simulink model "model3_19b"  (R2019b)
settings: Solver=VariableStepAuto  StartTime=0.0  StopTime=200  RelTol=1e-3
model workspace (MAT data in the model file):
  x2xx = 0
values from neighbouring files (symbols this model uses):
  axle_rate_limit = 1    [call_AFG4hil_s1v1.m]
  Kad = 0.0    (= 0)    [call_AFG4hil_s1v1.m]
  Kai = 0.05    [call_AFG4hil_s1v1.m]
  Kap = 0.1    [call_AFG4hil_s1v1.m]
  KDspd = 0.1    [call_AFG4hil_s1v1.m]    (also in call_AFG_s1v1.m = 0)
  KIspd = 0.1    [call_AFG4hil_s1v1.m]    (also in call_AFG_s1v1.m = 0)
  KPspd = 10    [call_AFG4hil_s1v1.m]    (also in call_AFG_s1v1.m = 20)
  Lspd = -7    [call_AFG4hil_s1v1.m]
  Nspd = 10    [call_AFG4hil_s1v1.m]
  Tmc = 0.02    [call_AFG4hil_s1v1.m]    (also in call_AFG_s1v1.m = 0.01)
  TRACK = temptrack    [article.m]    (also in calculate_offtrack.m; call_AFG4hil_s1v1.m = trackgen4(2,50); call_AFG_s1v1.m = trackgen4(2,50); tracktest.m)
  Tst = 0.05    [call_AFG4hil_s1v1.m]    (also in call_AFG_s1v1.m = 0.02)
  Uspd = 5    [call_AFG4hil_s1v1.m]
  vconst = 15*kph    (= 4.16666666667)    [call_AFG4hil_s1v1.m]    (also in call_AFG_s1v1.m = 5.55555555556)
undefined symbols (not defined in the file or in its folder): PARSa, PARSu, Q0
libraries: simulink x2
settings Model: Creator=DJW  LastModifiedBy=14668

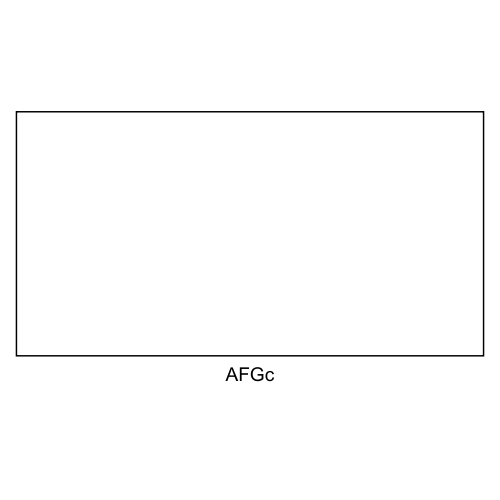
[thumbnail: Simulink's stored preview of the top-level diagram]
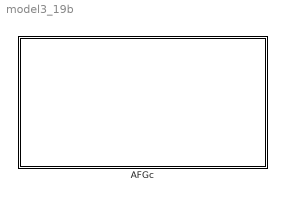
== system model3_19b ==
  AFGc : Subsystem

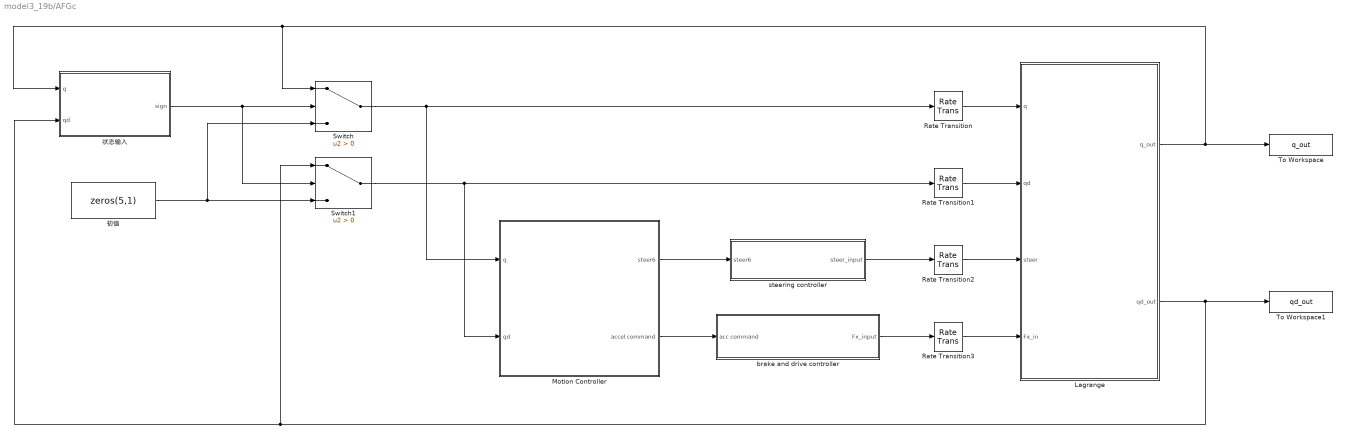
== system model3_19b/AFGc ==
  " Motion Controller" : Subsystem  SystemSampleTime=Tmc
  Lagrange : Subsystem
  Rate Transition{,1..3} (4 alike) : RateTransition
  Switch : Switch  Criteria=u2 > Threshold
  Switch1 : Switch  Criteria=u2 > Threshold
  To Workspace : ToWorkspace  VariableName=q_out  SampleTime=-1
  To Workspace1 : ToWorkspace  VariableName=qd_out  SampleTime=-1
  brake and drive controller : Subsystem
  steering controller : Subsystem
  初值 : Constant  Value=zeros(5,1)
  状态输入 : MATLAB Function  TreatAsAtomicUnit=on
  wires:
  " Motion Controller"/1(steer6) -> steering controller/1(steer6)
  " Motion Controller"/2(accel command) -> brake and drive controller/1(acc command)
  steering controller/1(steer_input) -> Rate Transition2/1
  brake and drive controller/1(Fx_input) -> Rate Transition3/1
  Lagrange/1(q_out) -> To Workspace/1, Switch/1, 状态输入/1(q)
  Lagrange/2(qd_out) -> To Workspace1/1, Switch1/1, 状态输入/2(qd)
  状态输入/1(sign) -> Switch1/2, Switch/2
  初值/1 -> Switch1/3, Switch/3
  Rate Transition2/1 -> Lagrange/3(steer)
  Rate Transition3/1 -> Lagrange/4(Fx_in)
  Rate Transition/1 -> Lagrange/1(q)
  Rate Transition1/1 -> Lagrange/2(qd)
  Switch1/1 -> " Motion Controller"/2(qd), Rate Transition1/1
  Switch/1 -> " Motion Controller"/1(q), Rate Transition/1

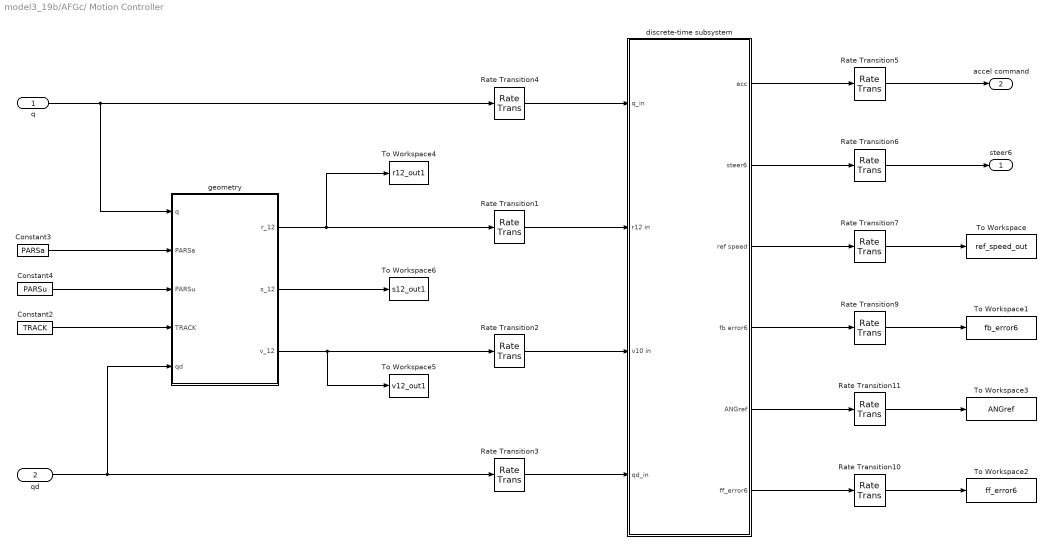
== system model3_19b/AFGc/ Motion Controller ==
  q : Inport
  qd : Inport  Port=2
  Constant2 : Constant  Value=TRACK
  Constant3 : Constant  Value=PARSa
  Constant4 : Constant  Value=PARSu
  Rate Transition{1..7,9..11} (10 alike) : RateTransition
  To Workspace : ToWorkspace  VariableName=ref_speed_out  SampleTime=-1
  To Workspace1 : ToWorkspace  VariableName=fb_error6  SampleTime=-1
  To Workspace2 : ToWorkspace  VariableName=ff_error6  SampleTime=-1
  To Workspace3 : ToWorkspace  VariableName=ANGref  SampleTime=-1
  To Workspace4 : ToWorkspace  VariableName=r12_out1  SampleTime=-1
  To Workspace5 : ToWorkspace  VariableName=v12_out1  SampleTime=-1
  To Workspace6 : ToWorkspace  VariableName=s12_out1  SampleTime=-1
  discrete-time subsystem : Subsystem  TreatAsAtomicUnit=on  SystemSampleTime=Tmc
  geometry : MATLAB Function  TreatAsAtomicUnit=on
  steer6 : Outport
  accel command : Outport  Port=2
  wires:
  q/1 -> geometry/1(q), Rate Transition4/1
  discrete-time subsystem/1(acc) -> Rate Transition5/1
  Rate Transition2/1 -> discrete-time subsystem/3(v10 in)
  Rate Transition4/1 -> discrete-time subsystem/1(q_in)
  Rate Transition5/1 -> accel command/1
  Rate Transition6/1 -> steer6/1
  qd/1 -> geometry/5(qd), Rate Transition3/1
  Rate Transition7/1 -> To Workspace/1
  discrete-time subsystem/3(ref speed) -> Rate Transition7/1
  Rate Transition9/1 -> To Workspace1/1
  Rate Transition10/1 -> To Workspace2/1
  discrete-time subsystem/5(ANGref) -> Rate Transition11/1
  Rate Transition11/1 -> To Workspace3/1
  Rate Transition3/1 -> discrete-time subsystem/4(qd_in)
  discrete-time subsystem/4(fb error6) -> Rate Transition9/1
  discrete-time subsystem/6(ff_error6) -> Rate Transition10/1
  Rate Transition1/1 -> discrete-time subsystem/2(r12 in)
  discrete-time subsystem/2(steer6) -> Rate Transition6/1
  Constant4/1 -> geometry/3(PARSu)
  geometry/3(v_12) -> To Workspace5/1, Rate Transition2/1
  geometry/2(s_12) -> To Workspace6/1
  geometry/1(r_12) -> To Workspace4/1, Rate Transition1/1
  Constant2/1 -> geometry/4(TRACK)
  Constant3/1 -> geometry/2(PARSa)

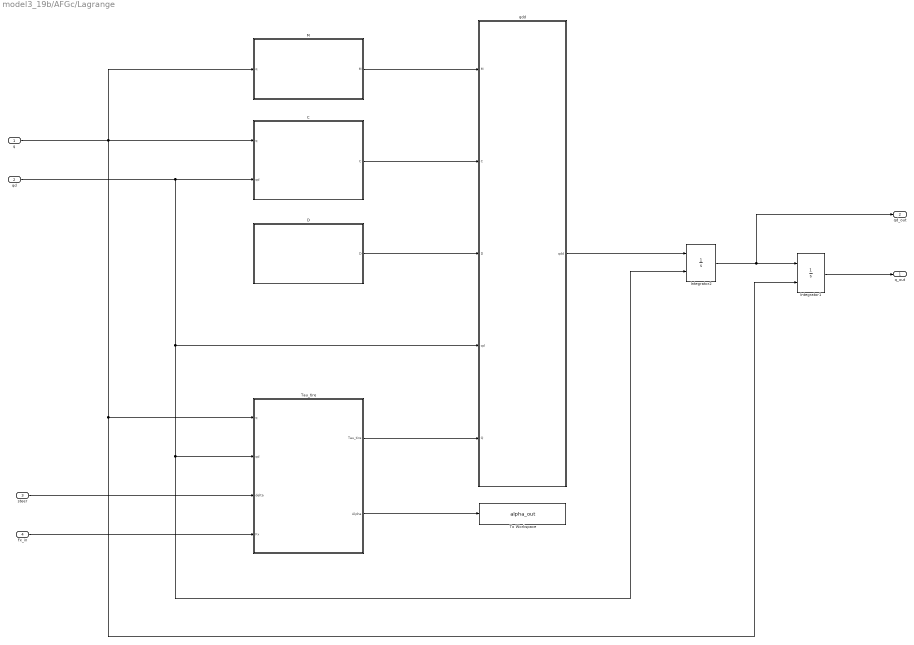
== system model3_19b/AFGc/Lagrange ==
  q : Inport
  qd : Inport  Port=2
  steer : Inport  Port=3
  Fx_in : Inport  Port=4
  C : MATLAB Function  TreatAsAtomicUnit=on
  D : MATLAB Function  TreatAsAtomicUnit=on
  Integrator1 : Integrator  InitialConditionSource=external  InitialCondition=Q0
  Integrator2 : Integrator  InitialConditionSource=external  InitialCondition=zeros(5,1)
  M : MATLAB Function  TreatAsAtomicUnit=on
  Tau_tire : MATLAB Function  TreatAsAtomicUnit=on
  To Workspace : ToWorkspace  VariableName=alpha_out  SampleTime=-1
  qdd : MATLAB Function  TreatAsAtomicUnit=on
  q_out : Outport
  qd_out : Outport  Port=2
  wires:
  Integrator1/1 -> q_out/1
  Fx_in/1 -> Tau_tire/4(Fx)
  q/1 -> Tau_tire/1(q), Integrator1/2, M/1(q), C/1(q)
  qd/1 -> Tau_tire/2(qd), Integrator2/2, qdd/4(qd), C/2(qd)
  steer/1 -> Tau_tire/3(delta)
  Tau_tire/2(Alpha) -> To Workspace/1
  qdd/1(qdd) -> Integrator2/1
  Integrator2/1 -> qd_out/1, Integrator1/1
  M/1(M) -> qdd/1(M)
  C/1(C) -> qdd/2(C)
  Tau_tire/1(Tau_tire) -> qdd/5(Q)
  D/1(D) -> qdd/3(D)

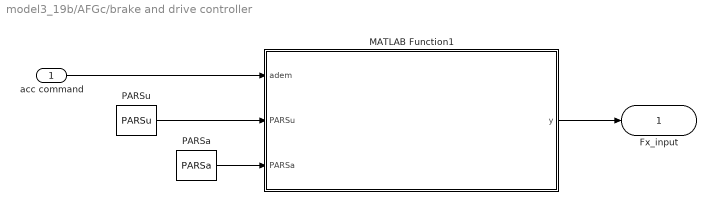
== system model3_19b/AFGc/brake and drive controller ==
  acc command : Inport
  " PARSu" : Constant  Value=PARSu
  MATLAB Function1 : MATLAB Function  TreatAsAtomicUnit=on
  PARSa : Constant  Value=PARSa
  Fx_input : Outport  VectorParamsAs1DForOutWhenUnconnected=off
  wires:
  PARSa/1 -> MATLAB Function1/3(PARSa)
  acc command/1 -> MATLAB Function1/1(adem)
  " PARSu"/1 -> MATLAB Function1/2(PARSu)
  MATLAB Function1/1(y) -> Fx_input/1

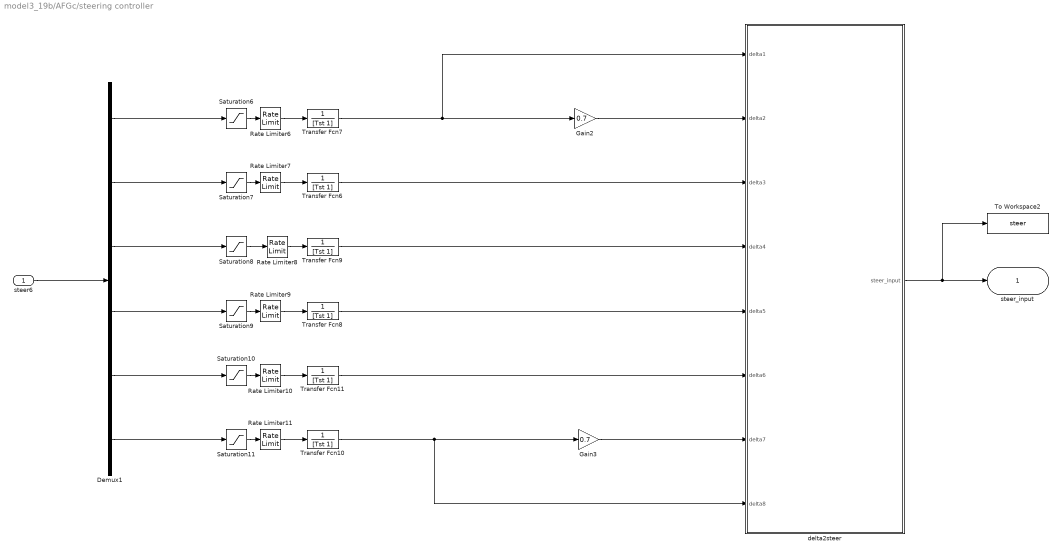
== system model3_19b/AFGc/steering controller ==
  steer6 : Inport
  Demux1 : Demux  Outputs=6
  Gain2 : Gain  Gain=0.7
  Gain3 : Gain  Gain=0.7
  Rate Limiter{6..11} (6 alike) : RateLimiter  RisingSlewLimit=3  FallingSlewLimit=-3  SampleTimeMode=inherited
  Saturation10 : Saturate  UpperLimit=0.3491  LowerLimit=-0.3491
  Saturation11 : Saturate  UpperLimit=0.2443  LowerLimit=-0.2443
  Saturation6 : Saturate  UpperLimit=0.3491  LowerLimit=-0.3491
  Saturation7 : Saturate  UpperLimit=0.2443  LowerLimit=-0.2443
  Saturation8 : Saturate  UpperLimit=0.3491  LowerLimit=-0.3491
  Saturation9 : Saturate  UpperLimit=0.2443  LowerLimit=-0.2443
  To Workspace2 : ToWorkspace  VariableName=steer  SampleTime=-1
  Transfer Fcn{6..11} (6 alike) : TransferFcn  Denominator=[Tst 1]
  delta2steer : MATLAB Function  TreatAsAtomicUnit=on
  steer_input : Outport
  wires:
  Demux1/2 -> Saturation7/1
  Saturation8/1 -> Rate Limiter8/1
  Rate Limiter9/1 -> Transfer Fcn8/1
  Transfer Fcn8/1 -> delta2steer/5(delta5)
  Rate Limiter11/1 -> Transfer Fcn10/1
  Transfer Fcn9/1 -> delta2steer/4(delta4)
  Demux1/4 -> Saturation9/1
  Demux1/1 -> Saturation6/1
  Transfer Fcn7/1 -> delta2steer/1(delta1), Gain2/1
  Saturation9/1 -> Rate Limiter9/1
  Saturation10/1 -> Rate Limiter10/1
  Rate Limiter7/1 -> Transfer Fcn6/1
  Demux1/5 -> Saturation10/1
  Rate Limiter10/1 -> Transfer Fcn11/1
  Rate Limiter6/1 -> Transfer Fcn7/1
  Saturation6/1 -> Rate Limiter6/1
  Saturation7/1 -> Rate Limiter7/1
  Demux1/3 -> Saturation8/1
  Saturation11/1 -> Rate Limiter11/1
  Demux1/6 -> Saturation11/1
  Transfer Fcn11/1 -> delta2steer/6(delta6)
  Transfer Fcn6/1 -> delta2steer/3(delta3)
  Rate Limiter8/1 -> Transfer Fcn9/1
  steer6/1 -> Demux1/1
  Transfer Fcn10/1 -> Gain3/1, delta2steer/8(delta8)
  Gain3/1 -> delta2steer/7(delta7)
  Gain2/1 -> delta2steer/2(delta2)
  delta2steer/1(steer_input) -> To Workspace2/1, steer_input/1

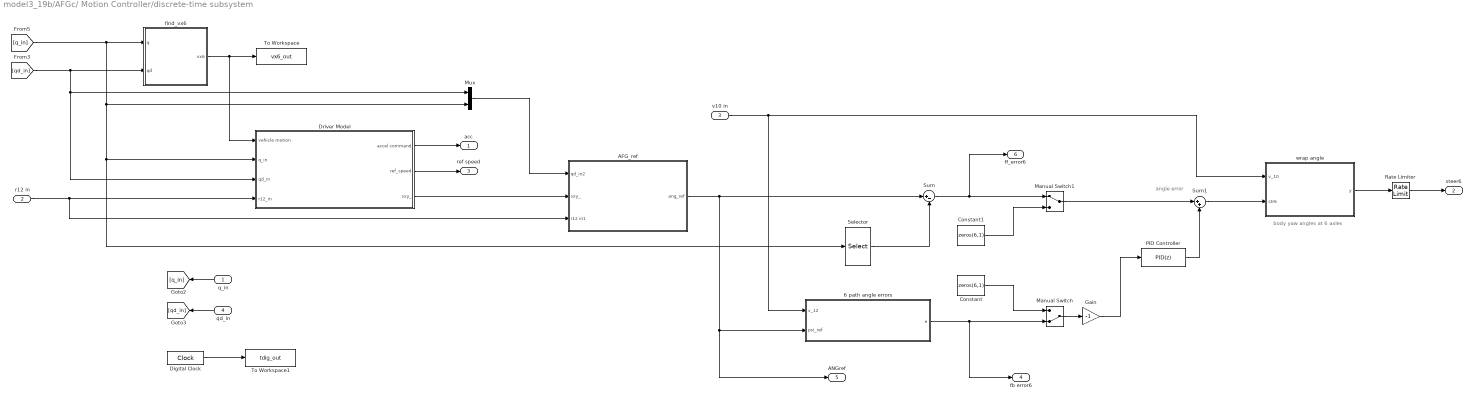
== system model3_19b/AFGc/ Motion Controller/discrete-time subsystem ==
  note: angle error
  note: body yaw
      | angles at 6 axles
  q_in : Inport
  r12 in : Inport  Port=2
  v10 in : Inport  Port=3
  qd_in : Inport  Port=4
  6 path angle errors : MATLAB Function  TreatAsAtomicUnit=on
  AFG_ref : Subsystem
  Constant : Constant  Value=zeros(6,1)
  Constant1 : Constant  Value=zeros(6,1)
  Digital Clock : DigitalClock  SampleTime=-1
  Driver Model : Subsystem  TreatAsAtomicUnit=on  SystemSampleTime=0.01
  Gain : Gain  Gain=-1
  Manual Switch : ManualSwitch  CurrentSetting=0
  Manual Switch1 : ManualSwitch
  Mux : Mux  Inputs=2
  PID Controller : simulink/Continuous/PID Controller  Controller=PID  Form=Parallel  TimeDomain=Discrete-time  SampleTime=-1  IntegratorMethod=Forward Euler  FilterMethod=Forward Euler  ControllerParametersSource=internal  P=Kap  I=Kai  D=Kad  N=100  UseFilter=off  TunerSelectOption=Transfer Function Based (PID Tuner App)  InitialConditionSource=internal  InitialConditionForIntegrator=0  InitialConditionForFilter=0  DifferentiatorICPrevScaledInput=0  ExternalReset=none  TrackingMode=off  Kt=1  LimitOutput=on  UpperSaturationLimit=0.1  LowerSaturationLimit=-0.1  LinearizeAsGain=on  AntiWindupMode=clamping  Kb=1  POutMin=[]  POutMax=[]  IOutMin=[]  IOutMax=[]  DOutMin=[]  DOutMax=[]  NOutMin=[]  NOutMax=[]  SumOutMin=[]  SumOutMax=[]  SaturationOutMin=[]  SaturationOutMax=[]  PParamMin=[]  PParamMax=[]  IParamMin=[]  IParamMax=[]  DParamMin=[]  DParamMax=[]  NParamMin=[]  NParamMax=[]  KbParamMin=[]  KbParamMax=[]  KtParamMin=[]  KtParamMax=[]  KbOutMin=[]  KbOutMax=[]  KtOutMin=[]  KtOutMax=[]  IntegratorOutMin=[]  IntegratorOutMax=[]  FilterOutMin=[]  FilterOutMax=[]  SumI1OutMin=[]  SumI1OutMax=[]  SumI2OutMin=[]  SumI2OutMax=[]  SumI3OutMin=[]  SumI3OutMax=[]  SumI4OutMin=[]  SumI4OutMax=[]  SumDOutMin=[]  SumDOutMax=[]  DifferentiatorOutMin=[]  DifferentiatorOutMax=[]  FilterDiffOutCoefMin=[]  FilterDiffOutCoefMax=[]  ReciprocalOutMin=[]  ReciprocalOutMax=[]  SumDenOutMin=[]  SumDenOutMax=[]  SumNumOutMin=[]  SumNumOutMax=[]  DivideOutMin=[]  DivideOutMax=[]  IntegratorContinuousStateAttributes=''  IntegratorStateMustResolveToSignalObject=off  IntegratorRTWStateStorageClass=Auto  FilterContinuousStateAttributes=''  FilterStateMustResolveToSignalObject=off  FilterRTWStateStorageClass=Auto  ParallelPVariant=InternalParameters  IdealPVariant=Disabled  IVariant=InternalParameters  DVariant=InternalParameters  IntegratorVariant=Discrete  SatVariant=Enabled  AWVariant=DiscClampingParallel  PCopyVariant=Disabled  TRVariant=Disabled  FdbkBlocksVariant=Forward  IdealPFdbkVariant=Disabled  SatFdbkVariant=Disabled  DerivativeFilterVariant=Differentiator  NVariant=Passthrough  NCopyVariant=Disabled_SignalSpec  FilterICVariant=InternalICsDifferentiator  IntegratorICVariant=InternalICs  ExternalResetVariant=Disabled  TRSumVariant=Passthrough  SumFdbkVariant=Disabled  SumVariant=Sum_PID
  Rate Limiter : RateLimiter  RisingSlewLimit=axle_rate_limit  FallingSlewLimit=-axle_rate_limit  SampleTimeMode=inherited
  Selector : Selector  InputPortWidth=5  IndexOptions=Index vector (dialog)  Indices=[3 3 4 4 5 5]  OutputSizes=1
  Sum : Sum  Inputs=|+-
  Sum1 : Sum  Inputs=|++
  To Workspace : ToWorkspace  VariableName=vx6_out  SampleTime=-1
  To Workspace1 : ToWorkspace  VariableName=tdig_out  SampleTime=-1
  find_vx6 : MATLAB Function  TreatAsAtomicUnit=on
  wrap angle : MATLAB Function  TreatAsAtomicUnit=on
  acc : Outport
  steer6 : Outport  Port=2
  ref speed : Outport  Port=3
  fb error6 : Outport  Port=4
  ANGref : Outport  Port=5
  ff_error6 : Outport  Port=6
  wires:
  Driver Model/1(accel command) -> acc/1
  q_in/1 -> [q_in]
  Gain/1 -> PID Controller/1
  qd_in/1 -> [qd_in]
  [q_in] -> Selector/1, Driver Model/2(q_in), Mux/2, find_vx6/1(q)
  Digital Clock/1 -> To Workspace1/1
  find_vx6/1(vx6) -> To Workspace/1, Driver Model/1(vehicle motion)
  [qd_in] -> Driver Model/3(qd_in), Mux/1, find_vx6/2(qd)
  Selector/1 -> Sum/2
  6 path angle errors/1(e) -> Manual Switch/2, fb error6/1
  wrap angle/1(y) -> Rate Limiter/1
  Sum/1 -> Manual Switch1/1, ff_error6/1
  Sum1/1 -> wrap angle/2(str6)
  v10 in/1 -> 6 path angle errors/1(v_12), wrap angle/1(v_10)
  Driver Model/2(ref_speed) -> ref speed/1
  Rate Limiter/1 -> steer6/1
  Manual Switch/1 -> Gain/1
  Constant/1 -> Manual Switch/1
  Constant1/1 -> Manual Switch1/2
  Mux/1 -> AFG_ref/1(qd_in2)
  r12 in/1 -> Driver Model/4(r12_in), AFG_ref/3(r12 in1)
  Driver Model/3(sxy_) -> AFG_ref/2(sxy_)
  Manual Switch1/1 -> Sum1/1
  PID Controller/1 -> Sum1/2
  AFG_ref/1(ang_ref) -> ANGref/1, 6 path angle errors/2(psi_ref), Sum/1

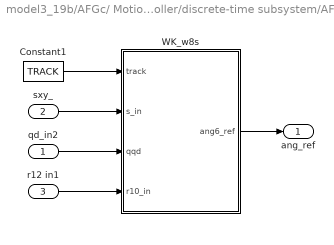
== system model3_19b/AFGc/ Motion Controller/discrete-time subsystem/AFG_ref ==
  qd_in2 : Inport
  sxy_ : Inport  Port=2
  r12 in1 : Inport  Port=3
  Constant1 : Constant  Value=TRACK
  WK_w8s : MATLAB Function  TreatAsAtomicUnit=on
  ang_ref : Outport
  wires:
  Constant1/1 -> WK_w8s/1(track)
  sxy_/1 -> WK_w8s/2(s_in)
  WK_w8s/1(ang6_ref) -> ang_ref/1
  qd_in2/1 -> WK_w8s/3(qqd)
  r12 in1/1 -> WK_w8s/4(r10_in)

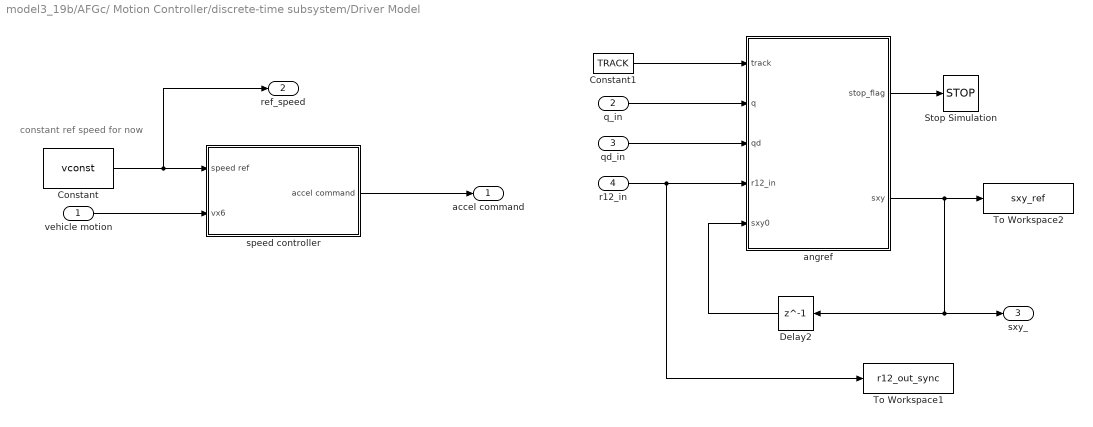
== system model3_19b/AFGc/ Motion Controller/discrete-time subsystem/Driver Model ==
  note: constant ref speed for now
  vehicle motion : Inport
  q_in : Inport  Port=2
  qd_in : Inport  Port=3
  r12_in : Inport  Port=4
  Constant : Constant  Value=vconst
  Constant1 : Constant  Value=TRACK
  Delay2 : Delay  DelayLength=1
  Stop Simulation : Stop
  To Workspace1 : ToWorkspace  VariableName=r12_out_sync  SampleTime=-1
  To Workspace2 : ToWorkspace  VariableName=sxy_ref  SampleTime=-1
  angref : MATLAB Function  TreatAsAtomicUnit=on
  speed controller : Subsystem
  accel command : Outport
  ref_speed : Outport  Port=2
  sxy_ : Outport  Port=3
  wires:
  qd_in/1 -> angref/3(qd)
  angref/1(stop_flag) -> Stop Simulation/1
  Constant1/1 -> angref/1(track)
  vehicle motion/1 -> speed controller/2(vx6)
  angref/2(sxy) -> sxy_/1, Delay2/1, To Workspace2/1
  Delay2/1 -> angref/5(sxy0)
  speed controller/1(accel command) -> accel command/1
  Constant/1 -> speed controller/1(speed ref), ref_speed/1
  q_in/1 -> angref/2(q)
  r12_in/1 -> angref/4(r12_in), To Workspace1/1

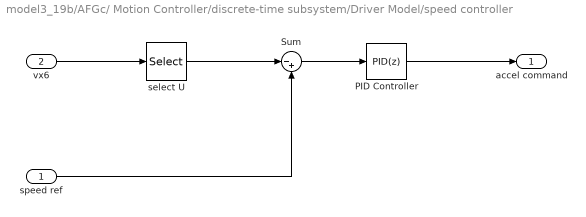
== system model3_19b/AFGc/ Motion Controller/discrete-time subsystem/Driver Model/speed controller ==
  speed ref : Inport
  vx6 : Inport  Port=2
  PID Controller : simulink/Continuous/PID Controller  Controller=PID  Form=Parallel  TimeDomain=Discrete-time  SampleTime=-1  IntegratorMethod=Forward Euler  FilterMethod=Forward Euler  ControllerParametersSource=internal  P=KPspd  I=KIspd  D=KDspd  N=Nspd  UseFilter=on  TunerSelectOption=Transfer Function Based (PID Tuner App)  InitialConditionSource=internal  InitialConditionForIntegrator=0  InitialConditionForFilter=0  DifferentiatorICPrevScaledInput=0  ExternalReset=none  TrackingMode=off  Kt=1  LimitOutput=on  UpperSaturationLimit=Uspd  LowerSaturationLimit=Lspd  LinearizeAsGain=on  AntiWindupMode=clamping  Kb=1  POutMin=[]  POutMax=[]  IOutMin=[]  IOutMax=[]  DOutMin=[]  DOutMax=[]  NOutMin=[]  NOutMax=[]  SumOutMin=[]  SumOutMax=[]  SaturationOutMin=[]  SaturationOutMax=[]  PParamMin=[]  PParamMax=[]  IParamMin=[]  IParamMax=[]  DParamMin=[]  DParamMax=[]  NParamMin=[]  NParamMax=[]  KbParamMin=[]  KbParamMax=[]  KtParamMin=[]  KtParamMax=[]  KbOutMin=[]  KbOutMax=[]  KtOutMin=[]  KtOutMax=[]  IntegratorOutMin=[]  IntegratorOutMax=[]  FilterOutMin=[]  FilterOutMax=[]  SumI1OutMin=[]  SumI1OutMax=[]  SumI2OutMin=[]  SumI2OutMax=[]  SumI3OutMin=[]  SumI3OutMax=[]  SumI4OutMin=[]  SumI4OutMax=[]  SumDOutMin=[]  SumDOutMax=[]  DifferentiatorOutMin=[]  DifferentiatorOutMax=[]  FilterDiffOutCoefMin=[]  FilterDiffOutCoefMax=[]  ReciprocalOutMin=[]  ReciprocalOutMax=[]  SumDenOutMin=[]  SumDenOutMax=[]  SumNumOutMin=[]  SumNumOutMax=[]  DivideOutMin=[]  DivideOutMax=[]  IntegratorContinuousStateAttributes=''  IntegratorStateMustResolveToSignalObject=off  IntegratorRTWStateStorageClass=Auto  FilterContinuousStateAttributes=''  FilterStateMustResolveToSignalObject=off  FilterRTWStateStorageClass=Auto  ParallelPVariant=InternalParameters  IdealPVariant=Disabled  IVariant=InternalParameters  DVariant=InternalParameters  IntegratorVariant=Discrete  SatVariant=Enabled  AWVariant=DiscClampingParallel  PCopyVariant=Disabled  TRVariant=Disabled  FdbkBlocksVariant=Forward  IdealPFdbkVariant=Disabled  SatFdbkVariant=Disabled  DerivativeFilterVariant=ForwardEulerFilter  NVariant=InternalParameters  NCopyVariant=Disabled  FilterICVariant=InternalICsFilter  IntegratorICVariant=InternalICs  ExternalResetVariant=Disabled  TRSumVariant=Passthrough  SumFdbkVariant=Disabled  SumVariant=Sum_PID
  Sum : Sum  Inputs=|-+
  select U : Selector  InputPortWidth=6  IndexOptions=Index vector (dialog)  Indices=[1]  OutputSizes=1
  accel command : Outport
  wires:
  Sum/1 -> PID Controller/1
  vx6/1 -> select U/1
  select U/1 -> Sum/1
  speed ref/1 -> Sum/2
  PID Controller/1 -> accel command/1

== matlab function model3_19b/AFGc/Lagrange/qdd ==
  data: M input; C input; D input; qd input; Q input; qdd output
function qdd = calculate_qdd(M, C, D, qd, Q)

qdd = inv(M)*(Q - C * qd - D * qd);

end

== matlab function model3_19b/AFGc/steering controller/delta2steer ==
  data: steer_input output; delta1 input; delta2 input; delta3 input; delta4 input; delta5 input; delta6 input; delta7 input; delta8 input
function steer_input = delta2Steer(delta1, delta2, delta3, delta4, delta5, delta6, delta7, delta8)

steer_input = zeros(8, 1);

steer_input(1) = delta1;
steer_input(2) = delta2;
steer_input(3) = delta3;
steer_input(4) = delta4;
steer_input(5) = delta5;
steer_input(6) = delta6;
steer_input(7) = delta7;
steer_input(8) = delta8;

end

== matlab function model3_19b/AFGc/ Motion Controller/discrete-time subsystem/6 path angle errors ==
  data: v_12 input; e output; psi_ref input
function e= compare_motions(v_12,psi_ref)
pa6=zeros(6,1); %path angles
refpts=[2,4,6,7,9,11]; %axle centres
v=[0,0];
for i=1:6
    j=refpts(i);
    v=v_12(j,:);
    pa6(i)=atan2(v(2),v(1));
end

e=wrap_angle(pa6-psi_ref);
end

== matlab function model3_19b/AFGc/Lagrange/Tau_tire ==
  data: q input; qd input; delta input; Fx input; Tau_tire output; Alpha output
function [Tau_tire, Alpha] = calculate_Tau_tire(q, qd, delta, Fx)

% coefficient

l_j1j2 = 11.4;
l_j2j3 = 9.4;
l_j1a1 = 2.5;
l_j1a2 = 4;
l_j1a3 = 9.9;
l_j2a4 = 1.5;
l_j2a5 = 7.9;
l_j3a6 = 1.5;
l_j3a7 = 7.4;
l_j3a8 = 8.9;

LL = [l_j1j2, l_j2j3, l_j1j2]';
JA = [l_j1a1, l_j1a2, l_j1a3, l_j2a4, l_j2a5, l_j3a6, l_j3a7, l_j3a8]';
XA = [l_j1j2, l_j1j2, l_j1j2, l_j2j3, l_j2j3, l_j1j2, l_j1j2, l_j1j2]' - JA;
IU = [1, 1, 1, 2, 2, 3, 3, 3]';

Ca = [3065 * 180 / pi, 3065 * 180 / pi, 3065 * 180 / pi, 3065 * 180 / pi, 3065 * 180 / pi, 3065 * 180 / pi, 3065 * 180 / pi, 3065 * 180 / pi]';

uu = zeros(2, 3);
nn = zeros(2, 3);
for i = 1:3
    uu(:, i)=[cos(q(i + 2)), sin(q(i + 2))]';
    nn(:, i)=[-sin(q(i + 2)), cos(q(i + 2))]';
end

psi1 = q(3);
psi2 = q(4);
psi3 = q(5);
xd = qd(1);
yd = qd(2);
psi1d = qd(3);
psi2d = qd(4);
psi3d = qd(5);
psij = [psi1, psi2, psi3]';
l_ja = [l_j1a1, l_j1a2, l_j1a3, l_j2a4, l_j2a5, l_j3a6, l_j3a7, l_j3a8]';

Rot_w2v = zeros(2, 2, 3);
for i = 1:3
    Rot_w2v(:, :, i) = [cos(psij(i)), -sin(psij(i));
                        sin(psij(i)), cos(psij(i));];
end

Rot_v2t = zeros(2, 2, 8);
for i = 1:8
    Rot_v2t(:, :, i) = [cos(delta(i)), -sin(delta(i));
                        sin(delta(i)), cos(delta(i));];
end

vxj = zeros(3, 1);
vyj = zeros(3, 1);
vxj(1) = xd;
vyj(1) = yd;
vxj(2) = xd + l_j1j2*sin(psi1)*psi1d;
vyj(2) = yd - l_j1j2*cos(psi1)*psi1d;
vxj(3) = xd + l_j1j2*sin(psi1)*psi1d + l_j2j3*sin(psi2)*psi2d;
vyj(3) = yd - l_j1j2*cos(psi1)*psi1d - l_j2j3*cos(psi2)*psi2d;
va = zeros(2, 8);
psidj = [psi1d, psi2d, psi3d]';
for i = 1:8
    va(:, i) = [vxj(IU(i)); vyj(IU(i))] - nn(:, IU(i))*l_ja(i)*psidj(IU(i));
end

Va_v = zeros(2, 8);  % axle velocities in locals
for i = 1:8
    Va_v(:, i) = inv(Rot_w2v(:, :, IU(i)))*va(:, i);
end

Fy = zeros(8, 1); 
Alpha = zeros(8, 1); 

beta = zeros(8, 1);
for i = 1:8
    beta(i) = atan2(Va_v(2, i), Va_v(1, i));
end

Vx_t = zeros(8, 1);
Vy_t = zeros(8, 1);
for i = 1:8
    Vx_t(i) = Va_v(1, i) * cos(delta(i)) + Va_v(2, i) * sin(delta(i));
    Vy_t(i) = -Va_v(1, i) * sin(delta(i)) + Va_v(2, i) * cos(delta(i));
end

for i = 1:8
    Alpha(i) = delta(i) - beta(i);
%     Fy(i) = -sign(Vy_t(i)) * Ca(i) * abs(Alpha(i));
    Fy(i) = Ca(i) * Alpha(i);
end

% for i = 1:8
%     vx = Va_v(1, i) * cos(delta(i)) + Va_v(2, i) * sin(delta(i));
%     vy = -Va_v(1, i) * sin(delta(i)) + Va_v(2, i) * cos(delta(i));
%     alpha = atan2(vy, vx);
%     Alpha(i) = alpha;
%     Fy(i) = -abs(Ca(i) * alpha) * sign(vy);
% end

L_long = [cos(psi1), cos(psi1), cos(psi1), cos(psi2), cos(psi2), cos(psi3), cos(psi3), cos(psi3);
           sin(psi1), sin(psi1), sin(psi1), sin(psi2), sin(psi2), sin(psi3), sin(psi3), sin(psi3);
           0, 0, 0, l_j1j2*sin(psi1-psi2), l_j1j2*sin(psi1-psi2), l_j1j2*sin(psi1-psi3), l_j1j2*sin(psi1-psi3), l_j1j2*sin(psi1-psi3);
           0, 0, 0, 0, 0, l_j2j3*sin(psi2-psi3), l_j2j3*sin(psi2-psi3), l_j2j3*sin(psi2-psi3);
           0, 0, 0, 0, 0, 0, 0, 0;];

L_lat = [-sin(psi1), -sin(psi1), -sin(psi1), -sin(psi2), -sin(psi2), -sin(psi3), -sin(psi3), -sin(psi3);
          cos(psi1), cos(psi1), cos(psi1), cos(psi2), cos(psi2), cos(psi3), cos(psi3), cos(psi3);
          -l_j1a1, -l_j1a2, -l_j1a3, -l_j1j2*cos(psi1-psi2), -l_j1j2*cos(psi1-psi2), -l_j1j2*cos(psi1-psi3), -l_j1j2*cos(psi1-psi3), -l_j1j2*cos(psi1-psi3);
          0, 0, 0, -l_j2a4, -l_j2a5, -l_j2j3*cos(psi2-psi3), -l_j2j3*cos(psi2-psi3), -l_j2j3*cos(psi2-psi3);
          0, 0, 0, 0, 0, -l_j3a6, -l_j3a7, -l_j3a8;];

Delta_c = zeros(8, 8);
Delta_s = zeros(8, 8);
for i = 1:8
    Delta_c(i, i) = cos(delta(i));
    Delta_s(i, i) = sin(delta(i));
end

Tau_tire = L_long * (Delta_c * Fx - Delta_s * Fy) + L_lat * (Delta_s * Fx + Delta_c * Fy);

end

== matlab function model3_19b/AFGc/状态输入 ==
  data: q input; sign output; qd input
function sign = is_start(q, qd)

sign = 1;
if q == zeros(5,1) 
    if qd == zeros(5,1)
        sign = 0;
    end
end

end

== matlab function model3_19b/AFGc/ Motion Controller/geometry ==
  settings: updateMethod=DISCRETE
  data: r_12 output; s_12 output; q input; PARSa input; PARSu input; TRACK input; qd input; v_12 output
function [r_12,s_12,v_12] = ART_geom4(q,PARSa,PARSu, TRACK, qd)

LL=PARSu(:,3);
XX1=LL(1)-PARSa(1:3,1);
XX2=LL(2)-PARSa(4:5,1);
XX3=LL(3)-PARSa(6:8,1);
u1=[cos(q(3));sin(q(3))];n1=[-sin(q(3));cos(q(3))];
u2=[cos(q(4));sin(q(4))];n2=[-sin(q(4));cos(q(4))];
u3=[cos(q(5));sin(q(5))];n3=[-sin(q(5));cos(q(5))];


%% % rij for key points on ART, i for unit and j for axle (i=0 for joints, inlcuding the virtual one)
r01=q(1:2); %front (virtual) joint, 1
r11=r01-XX1(1)*u1;
r12=r01-XX1(2)*u1;
r13=r01-XX1(3)*u1;
r02=r01-LL(1)*u1;%joint, 2
r21=r02-XX2(1)*u2;
r22=r02-XX2(2)*u2;
r03=r02-LL(2)*u2;
r31=r03-XX3(1)*u3;
r32=r03-XX3(2)*u3;
r33=r03-XX3(3)*u3;
r04=r03-LL(3)*u3;
r_12=[r01,r11,r12,r13,r02,r21,r22,r03,r31,r32,r33,r04]';

v01=qd(1:2);
v11=v01-qd(3)*XX1(1)*n1;
v12=v01-qd(3)*XX1(2)*n1;
v13=v01-qd(3)*XX1(3)*n1;
v02=v01-qd(3)*LL(1)*n1;
v21=v02-qd(4)*XX2(1)*n2;
v22=v02-qd(4)*XX2(2)*n2;
v03=v02-qd(4)*LL(2)*n2;
v31=v03-qd(5)*XX3(1)*n3;
v32=v03-qd(5)*XX3(2)*n3;
v33=v03-qd(5)*XX3(3)*n3;
v04=v03-qd(5)*LL(3)*n3;
v_12=[v01,v11,v12,v13,v02,v21,v22,v03,v31,v32,v33,v04]';

s_12=zeros(12,2);
for i=1:12
    x=r_12(i,:);
    sxy=x2s(x,TRACK); % track coordinates
    s_12(i,:)=sxy;
end

end

== matlab function model3_19b/AFGc/ Motion Controller/discrete-time subsystem/Driver Model/angref ==
  data: stop_flag output; track input; q input; qd input; r12_in input; sxy0 input; sxy output
function [stop_flag,sxy] = ssav(track,q,qd, r12_in,sxy0)


sxy=[0 0]'; %send as vector
stop_flag=0;
spd=hypot(qd(1),qd(2));

% x=[q(1),q(2)]; % location of front joint, row vector
x=r12_in(5,:);
if spd<0.1
    ss=x2s(x,track);
else
    ss=x2ss(x,track,sxy0(1),20);%tolerance set to be 20
end
sxy=[ss(1);ss(2)];


if track(end,1)-ss(1) < 25
    disp('simulation stopped near end of track')
    stop_flag=1; 
end

return

== matlab function model3_19b/AFGc/Lagrange/D ==
  data: D output
function D = calculate_D()

d1 = 0;
d2 = 0;

delta_kj = eye(3);
dj = [0, d1, d2, 0]';
D = zeros(5);

for k = 1:5
    for l = 1:5
        if k > 2 && l > 2
            if  l == k
                D(k, l) = (1 - delta_kj(1, k-2))*dj(k - 2) + (1 - delta_kj(3, k-2))*dj(k - 1);
            elseif l == k-1
                D(k, l) = -(1 - delta_kj(1, k-2))*dj(k - 2);
            elseif l == k+1
                D(k, l) = -(1 - delta_kj(3, k-2))*dj(k - 1);
            else
                D(k, l) = 0;
            end
        end
    end
end

end

== matlab function model3_19b/AFGc/ Motion Controller/discrete-time subsystem/wrap angle ==
  data: v_10 input; str6 input; y output
function y = wrap_steer_angle(v_10,str6)
%#codegen


y=wrap_angle(str6(1:6));
% y=zeros(5,1);
end

== matlab function model3_19b/AFGc/brake and drive controller/MATLAB Function1 ==
  data: adem input; y output; PARSu input; PARSa input
function y = wheel_force_distibution(adem,PARSu,PARSa)

y=zeros(8,1); 
mass=sum(PARSu(:,1));
Na=size(PARSa,1);
if adem>0
    y(1:Na)=PARSa(:,4); %drive axle distribution
else
    y(1:Na)=PARSa(:,5); %brake force distribution
end
n=sum(y);
y=y*mass*adem/n;
end

== matlab function model3_19b/AFGc/Lagrange/C ==
  data: q input; qd input; C output
function C = calculate_C(q, qd)

m1 = 11142;
m3 = 11142;
m2 = 7651; 
l_j1j2 = 11.4;
l_j2j3 = 9.4;
l_j1g1 = 5.862; 
l_j2g2 = 4.643; 
l_j3g3 = 5.538; 

psi1 = q(3);
psi2 = q(4);
psi3 = q(5);
xd = qd(1);
yd = qd(2);
psi1d = qd(3);
psi2d = qd(4);
psi3d = qd(5);

C = [0, 0, (l_j1g1*m1 + l_j1j2*(m2 + m3))*cos(psi1)*psi1d, (l_j2g2*m2 + l_j2j3*m3)*cos(psi2)*psi2d, l_j3g3*m3*cos(psi3)*psi3d;
     0, 0, (l_j1g1*m1 + l_j1j2*(m2 + m3))*sin(psi1)*psi1d, (l_j2g2*m2 + l_j2j3*m3)*sin(psi2)*psi2d, l_j3g3*m3*sin(psi3)*psi3d;
     1/2*(l_j1g1*m1 + l_j1j2*(m2 + m3))*cos(psi1)*psi1d, 1/2*(l_j1g1*m1 + l_j1j2*(m2 + m3))*sin(psi1)*psi1d, -1/2*(l_j1g1*m1 + l_j1j2*(m2 + m3))*(xd*cos(psi1)+yd*sin(psi1))+1/2*(l_j2g2*l_j1j2*m2+l_j1j2*l_j2j3*m3)*sin(psi1-psi2)*psi2d+1/2*l_j3g3*l_j1j2*m3*sin(psi1-psi3)*psi3d, (l_j2g2*l_j1j2*m2+l_j1j2*l_j2j3*m3)*sin(psi1-psi2)*(-1/2*psi1d+psi2d), l_j3g3*l_j1j2*m3*sin(psi1-psi3)*(-1/2*psi1d+psi3d);
     1/2*(l_j2g2*m2 + l_j2j3*m3)*cos(psi2)*psi2d, 1/2*(l_j2g2*m2 + l_j2j3*m3)*sin(psi2)*psi2d, (l_j2g2*l_j1j2*m2+l_j1j2*l_j2j3*m3)*sin(psi1-psi2)*(-psi1d+1/2*psi2d), -1/2*(l_j2g2*m2+l_j2j3*m3)*(xd*cos(psi2)+yd*sin(psi2))-1/2*(l_j2g2*l_j1j2*m2+l_j1j2*l_j2j3*m3)*sin(psi1-psi2)*psi1d+1/2*l_j3g3*l_j2j3*m3*sin(psi2-psi3)*psi3d, l_j3g3*l_j2j3*m3*sin(psi2-psi3)*(-1/2*psi2d+psi3d);
     1/2*l_j3g3*m3*cos(psi3)*psi3d, 1/2*l_j3g3*m3*sin(psi3)*psi3d, l_j3g3*l_j1j2*m3*sin(psi1-psi3)*(-psi1d+1/2*psi3d), l_j3g3*l_j2j3*m3*sin(psi2-psi3)*(-psi2d+1/2*psi3d), -1/2*l_j3g3*m3*(xd*cos(psi3)+yd*sin(psi3))-1/2*l_j3g3*l_j1j2*m3*sin(psi1-psi3)*psi1d-1/2*l_j3g3*l_j2j3*m3*sin(psi2-psi3)*psi2d;];

end

== matlab function model3_19b/AFGc/ Motion Controller/discrete-time subsystem/find_vx6 ==
  settings: updateMethod=DISCRETE
  data: vx6 output; q input; qd input
function vx6 = vx_conversion(q,qd)
%#codegen
% convert q and qd to vx6 needed for the driver model

xxp=2; %nominal point P of driver 
u1=[cos(q(3));sin(q(3))];n1=[-sin(q(3));cos(q(3))];
rp = q(1:2)-xxp*u1;

v00=qd(1:2); %global velocity at front joint
vp=v00-qd(3)*xxp*n1; %move to driver point
U=dot(vp,u1);V=dot(vp,n1); %components in body axes (unit 1)
vx6=[U;V;qd(3);rp;q(3)]; %standard format ... [U,V,r,x,y,psi]'
end

== matlab function model3_19b/AFGc/ Motion Controller/discrete-time subsystem/AFG_ref/WK_w8s ==
  data: track input; ang6_ref output; s_in input; qqd input; r10_in input
function ang6_ref   = WK(track,s_in,qqd, r10_in)
% generate angref6 based on pure AFG, i.e., flow generated directly based
% on r6 out of r12

ang6_ref=zeros(6,1); 

q=qqd(1:5);qd=qqd(6:10);
spd=norm(qd(1:2));

r=zeros(6,2);
r(1,:)=r10_in(2,:);
r(2,:)=r10_in(4,:);
r(3,:)=r10_in(6,:);
r(4,:)=r10_in(7,:);
r(5,:)=r10_in(9,:);
r(6,:)=r10_in(11,:);

a_flow=0.5;
U0=1;

for i=1:6
    WC=complex(zeros(1,1)); %complex form of w
    [w,~]=w8s(r(i,:),track,spd,s_in(1),a_flow,U0);
    WC=w(1)+1i*w(2);
    if spd<0.1
        ang6_ref(i)=0;
    else
        ang6_ref(i)=angle(WC);
    end

end

return

== matlab function model3_19b/AFGc/Lagrange/M ==
  data: M output; q input
function M = calculate_M(q)

psi1 = q(3);
psi2 = q(4);
psi3 = q(5);

m1 = 11142;
m3 = 11142;
m2 = 7651; 
l_j1j2 = 11.4;
l_j2j3 = 9.4;
l_j1g1 = 5.862; 
l_j2g2 = 4.643; 
l_j3g3 = 5.538; 
iz1 = 143570; 
iz3 = 143570; 
iz2 = 37800;

l_kj = [l_j1g1, l_j1j2, l_j1j2;
             0, l_j2g2, l_j2j3;
             0,      0, l_j3g3;];
delta_kj = eye(3);
Jc = zeros(3, 5, 3);
for j = 1:3
    Jc(:, :, j) = [1, 0,  l_kj(1, j) * sin(psi1),  l_kj(2, j) * sin(psi2),  l_kj(3, j) * sin(psi3);
          0, 1, -l_kj(1, j) * cos(psi1), -l_kj(2, j) * cos(psi2), -l_kj(3, j) * cos(psi3);
          0, 0,          delta_kj(1, j),          delta_kj(2, j),          delta_kj(3, j);];
end

mj = [m1, m2, m3]';
izj = [iz1, iz2, iz3]';
Mj = zeros(3, 3, 3);
for j = 1:3
    Mj(:, :, j) = diag([mj(j), mj(j), izj(j)]);
end

M = zeros(5, 5);
for j = 1:3
    M = M + Jc(:, :, j)' * Mj(:, :, j) * Jc(:, :, j);
end

end
